simulink model "lookupTableDynamic_TestGen38"  (R2017b)
settings: Solver=FixedStepDiscrete  StartTime=0.0  StopTime=10.0  RelTol=1e-3
libraries: simulink x1
settings Model: Creator=ktrinh  LastModifiedBy=ktrinh
settings DebuggingCC: ParameterOverflowMsg=none

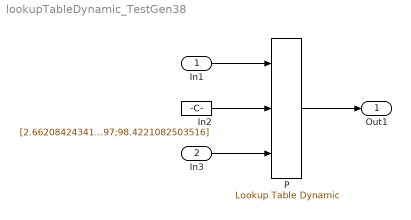
== system lookupTableDynamic_TestGen38 ==
  In1 : Inport  OutMin=0.66208  OutMax=100  OutDataTypeStr=uint16  PortDimensions=3
  In3 : Inport  Port=2  PortDimensions=5
  In2 : Constant  Value=[2.66208424341428;10.8198813861002;73.9083959262094;90.3654022115197;98.4221082503516]  OutDataTypeStr=uint16
  P : simulink/Lookup Tables/Lookup Table Dynamic  LookUpMeth=Use Input Above  OutDataType=fixdt('single')  OutScaling=[]  OutputDataTypeScalingMode=Specify via dialog  OutDataTypeStr=single  RndMeth=Nearest  DoSatur=off
      settings: SourceProductName=Simulink
  Out1 : Outport
  wires:
  In1/1 -> P/1
  In2/1 -> P/2
  In3/1 -> P/3
  P/1 -> Out1/1
